simulink model "assign1ol"  (Simulink 8.6)
settings: Solver=ode45  StartTime=0.0  StopTime=120.0  RelTol=1e-3
settings Model: Creator=AartsRGKM  LastModifiedBy=AartsRGKM
settings DataIOCC: SignalLoggingName=sigsOut
settings OptimizationCC: ExpressionDepthLimit=128
settings DebuggingCC: SaveWithParameterizedLinksMsg=none  SignalResolutionControl=TryResolveAllWithWarning  SolverPrmCheckMsg=none  MultiTaskDSMMsg=warning  MultiTaskCondExecSysMsg=none  FcnCallInpInsideContextMsg=EnableAllAsError  StateNameClashWarn=none
settings HardwareCC: TargetUnknown=on
settings GRTTargetCC: GeneratePreprocessorConditionals=Use local settings

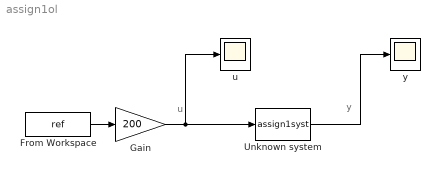
== system assign1ol ==
  note: u
  note: y
  From Workspace : FromWorkspace  VariableName=ref  SampleTime=0.01  Interpolate=off  OutputAfterFinalValue=Cyclic repetition
  Gain : Gain  Gain=200  SaturateOnIntegerOverflow=on  OutDataTypeStr=Inherit: Same as input  ParamDataTypeStr=Inherit: Same as input
  Unknown system : M-S-Function  FunctionName=assign1syst
  u : Scope
  y : Scope
  wires:
  From Workspace/1 -> Gain/1
  Unknown system/1 -> y/1
  Gain/1 -> Unknown system/1, u/1
